simulink model "Motor_Dynamics"  (R2026a)
settings: Solver=VariableStepAuto  StopTime=10
InitFcn:
  | Motor_dynamics_init
values from neighbouring files (symbols this model uses):
  b_m = 1.5e-4    (= 0.00015)    [Motor_Dynamics_TF.m]    (also in Motor_dynamics_init.m = 2.415e-06)
  J_m = 5e-5    (= 5e-05)    [Motor_Dynamics_TF.m]    (also in Motor_dynamics_init.m = 6.5e-07)
  K_emf = 0.025    [Motor_Dynamics_TF.m]    (also in Motor_dynamics_init.m = 0.00255)
  K_t = 0.025    [Motor_Dynamics_TF.m]    (also in Motor_dynamics_init.m = 0.00255)
  L = 0.002    [Motor_Dynamics_TF.m]    (also in Motor_dynamics_init.m = 0.000117)
  R = 0.6    [Motor_Dynamics_TF.m]    (also in Motor_dynamics_init.m = 0.117)
settings Model: Creator=Umesh  LastModifiedBy=Umesh

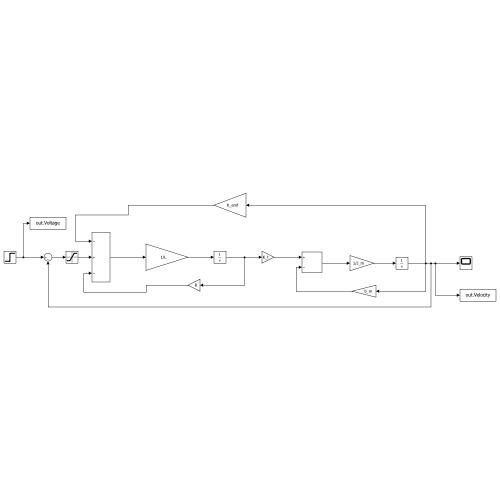
[thumbnail: Simulink's stored preview of the top-level diagram]
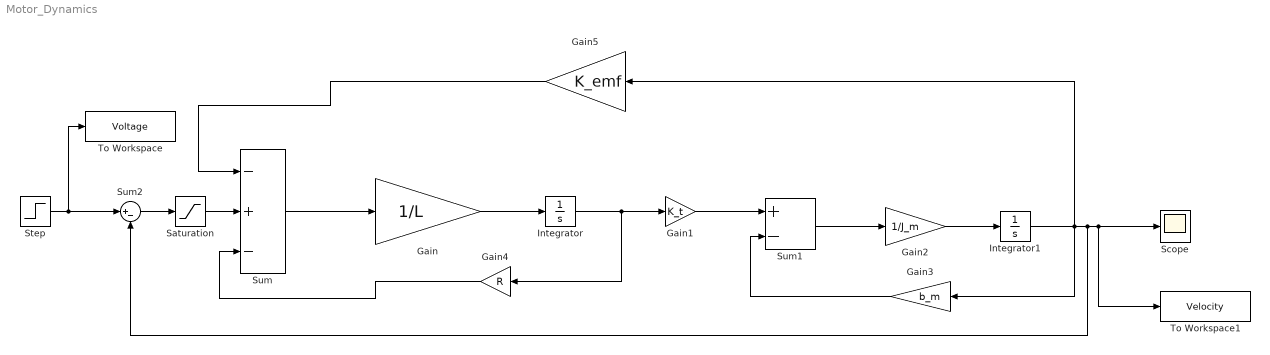
== system Motor_Dynamics ==
  Gain : Gain  Gain=1/L
  Gain1 : Gain  Gain=K_t
  Gain2 : Gain  Gain=1/J_m
  Gain3 : Gain  Gain=b_m
  Gain4 : Gain  Gain=R
  Gain5 : Gain  Gain=K_emf
  Integrator : Integrator
  Integrator1 : Integrator
  Saturation : Saturate  UpperLimit=12  LowerLimit=0
  Scope : Scope
      settings: ActiveDisplayYMinimum=-54.588872048135386  ActiveDisplayYMaximum=1645.93591666766  YLabel=Omega
  Step : Step  FinalValue=1000  SampleTime=0
  Sum : Sum  Inputs=-+-
  Sum1 : Sum  Inputs=+-
  Sum2 : Sum  Inputs=|+-
  To Workspace : ToWorkspace  VariableName=Voltage  SaveFormat=Timeseries  SampleTime=-1
  To Workspace1 : ToWorkspace  VariableName=Velocity  SaveFormat=Timeseries  SampleTime=-1
  wires:
  Sum/1 -> Gain/1
  Gain/1 -> Integrator/1
  Integrator/1 -> Gain4/1, Gain1/1
  Gain1/1 -> Sum1/1
  Sum1/1 -> Gain2/1
  Gain2/1 -> Integrator1/1
  Integrator1/1 -> Gain5/1, Gain3/1, Sum2/2, To Workspace1/1, Scope/1
  Gain3/1 -> Sum1/2
  Gain4/1 -> Sum/3
  Gain5/1 -> Sum/1
  Step/1 -> Sum2/1, To Workspace/1
  Saturation/1 -> Sum/2
  Sum2/1 -> Saturation/1
